simulink model "model"  (R2014a)
(part 3 of 3)

  _CN_133263110_220000_CN_163640749_220000/LConn3 -- T_133263110_220000_Няндома/LConn3 -- _CN_133263110_220000_CN_96836497_220000/LConn3 -- _CN_133263110_220000_CN_147416198_220000/LConn3 -- bus111/LConn1
  _CN_133263110_220000_CN_163640749_220000/RConn1 -- T_163640749_220000_Плесецк/LConn1 -- Плесецк___Новая_2_цепь_CN_163640749_220000_CN_124601500_220000/LConn1
  _CN_133263110_220000_CN_163640749_220000/RConn2 -- T_163640749_220000_Плесецк/LConn2 -- Плесецк___Новая_2_цепь_CN_163640749_220000_CN_124601500_220000/LConn2
  _CN_133263110_220000_CN_163640749_220000/RConn3 -- T_163640749_220000_Плесецк/LConn3 -- Плесецк___Новая_2_цепь_CN_163640749_220000_CN_124601500_220000/LConn3 -- bus112/LConn1
  _CN_133263110_220000_CN_96836497_220000/RConn1 -- T_96836497_220000_Коноша/LConn1 -- _CN_52300555_220000_CN_96836497_220000/LConn1
  _CN_133263110_220000_CN_96836497_220000/RConn2 -- T_96836497_220000_Коноша/LConn2 -- _CN_52300555_220000_CN_96836497_220000/LConn2
  _CN_133263110_220000_CN_96836497_220000/RConn3 -- T_96836497_220000_Коноша/LConn3 -- _CN_52300555_220000_CN_96836497_220000/LConn3 -- bus113/LConn1
  _CN_133263110_220000_CN_147416198_220000/RConn1 -- T_147416198_220000_Подстанция_220_кВ_«Вельск»/LConn1 -- Вельск___Шангалы_CN_147416198_220000_CN_265498319_220000/LConn1
  _CN_133263110_220000_CN_147416198_220000/RConn2 -- T_147416198_220000_Подстанция_220_кВ_«Вельск»/LConn2 -- Вельск___Шангалы_CN_147416198_220000_CN_265498319_220000/LConn2
  _CN_133263110_220000_CN_147416198_220000/RConn3 -- T_147416198_220000_Подстанция_220_кВ_«Вельск»/LConn3 -- Вельск___Шангалы_CN_147416198_220000_CN_265498319_220000/LConn3 -- bus114/LConn1
  _CN_52300555_220000_CN_331268073_220000/LConn1 -- "T_52300555__ПС_500кВ_\"Вологодская\""/LConn1 -- _CN_52300555_220000_CN_331298845_220000/LConn1 -- _CN_52300555_220000_CN_96836497_220000/RConn1 -- _CN_52300555_220000_CN_197906665_220000/LConn1 -- _CN_52300555_220000_CN_315281956_220000/LConn1
  _CN_52300555_220000_CN_331268073_220000/LConn2 -- "T_52300555__ПС_500кВ_\"Вологодская\""/LConn2 -- _CN_52300555_220000_CN_331298845_220000/LConn2 -- _CN_52300555_220000_CN_96836497_220000/RConn2 -- _CN_52300555_220000_CN_197906665_220000/LConn2 -- _CN_52300555_220000_CN_315281956_220000/LConn2
  _CN_52300555_220000_CN_331268073_220000/LConn3 -- "T_52300555__ПС_500кВ_\"Вологодская\""/LConn3 -- _CN_52300555_220000_CN_331298845_220000/LConn3 -- _CN_52300555_220000_CN_96836497_220000/RConn3 -- _CN_52300555_220000_CN_197906665_220000/LConn3 -- _CN_52300555_220000_CN_315281956_220000/LConn3 -- bus115/LConn1
  T_331268073_220000_ГПП_2/LConn1 -- _CN_52300555_220000_CN_331268073_220000/RConn1
  T_331268073_220000_ГПП_2/LConn2 -- _CN_52300555_220000_CN_331268073_220000/RConn2
  _CN_52300555_220000_CN_331268073_220000/RConn3 -- T_331268073_220000_ГПП_2/LConn3 -- bus116/LConn1
  T_331298845_220000_Явенга_тяговая/LConn1 -- _CN_52300555_220000_CN_331298845_220000/RConn1
  T_331298845_220000_Явенга_тяговая/LConn2 -- _CN_52300555_220000_CN_331298845_220000/RConn2
  _CN_52300555_220000_CN_331298845_220000/RConn3 -- T_331298845_220000_Явенга_тяговая/LConn3 -- bus117/LConn1
  T_197906665_220000_Кадниковский_тяговая/LConn1 -- _CN_52300555_220000_CN_197906665_220000/RConn1
  T_197906665_220000_Кадниковский_тяговая/LConn2 -- _CN_52300555_220000_CN_197906665_220000/RConn2
  _CN_52300555_220000_CN_197906665_220000/RConn3 -- T_197906665_220000_Кадниковский_тяговая/LConn3 -- bus118/LConn1
  T_315281956_220000_Сокол/LConn1 -- _CN_52300555_220000_CN_315281956_220000/RConn1
  T_315281956_220000_Сокол/LConn2 -- _CN_52300555_220000_CN_315281956_220000/RConn2
  _CN_52300555_220000_CN_315281956_220000/RConn3 -- T_315281956_220000_Сокол/LConn3 -- bus119/LConn1
  T_124601500_220000_Новая/LConn1 -- Плесецк___Новая_2_цепь_CN_163640749_220000_CN_124601500_220000/RConn1
  T_124601500_220000_Новая/LConn2 -- Плесецк___Новая_2_цепь_CN_163640749_220000_CN_124601500_220000/RConn2
  Плесецк___Новая_2_цепь_CN_163640749_220000_CN_124601500_220000/RConn3 -- T_124601500_220000_Новая/LConn3 -- bus120/LConn1
  Синдор___Микунь_CN_212471066_220000_CN_211036038_220000/RConn1 -- T_211036038_220000_Микунь/LConn1 -- _CN_276250552_220000_CN_211036038_220000/LConn1 -- Микунь___Сыктывкар_CN_217498367_220000_CN_211036038_220000/LConn1
  Синдор___Микунь_CN_212471066_220000_CN_211036038_220000/RConn2 -- T_211036038_220000_Микунь/LConn2 -- _CN_276250552_220000_CN_211036038_220000/LConn2 -- Микунь___Сыктывкар_CN_217498367_220000_CN_211036038_220000/LConn2
  Синдор___Микунь_CN_212471066_220000_CN_211036038_220000/RConn3 -- T_211036038_220000_Микунь/LConn3 -- _CN_276250552_220000_CN_211036038_220000/LConn3 -- Микунь___Сыктывкар_CN_217498367_220000_CN_211036038_220000/LConn3 -- bus121/LConn1
  "T_116869794_220000_Подстанция_\"Парголово\""/LConn1 -- _CN_116869794_220000_CN_23549613_220000/LConn1
  "T_116869794_220000_Подстанция_\"Парголово\""/LConn2 -- _CN_116869794_220000_CN_23549613_220000/LConn2
  _CN_116869794_220000_CN_23549613_220000/LConn3 -- "T_116869794_220000_Подстанция_\"Парголово\""/LConn3 -- bus122/LConn1
  "T_23549613_220000_Подстанция_\"Приморская\""/LConn1 -- _CN_116869794_220000_CN_23549613_220000/RConn1
  "T_23549613_220000_Подстанция_\"Приморская\""/LConn2 -- _CN_116869794_220000_CN_23549613_220000/RConn2
  _CN_116869794_220000_CN_23549613_220000/RConn3 -- "T_23549613_220000_Подстанция_\"Приморская\""/LConn3 -- bus123/LConn1
  T_105535524_220000_Промысловая/LConn1 -- Усинская___Промысловая_CN_105535524_220000_CN_105528914_220000/RConn1
  T_105535524_220000_Промысловая/LConn2 -- Усинская___Промысловая_CN_105535524_220000_CN_105528914_220000/RConn2
  Усинская___Промысловая_CN_105535524_220000_CN_105528914_220000/RConn3 -- T_105535524_220000_Промысловая/LConn3 -- bus124/LConn1
  Вельск___Шангалы_CN_147416198_220000_CN_265498319_220000/RConn1 -- T_265498319_220000_Шангалы/LConn1 -- Кизема__Шангалы_CN_163253148_220000_CN_265498319_220000/LConn1
  Вельск___Шангалы_CN_147416198_220000_CN_265498319_220000/RConn2 -- T_265498319_220000_Шангалы/LConn2 -- Кизема__Шангалы_CN_163253148_220000_CN_265498319_220000/LConn2
  Вельск___Шангалы_CN_147416198_220000_CN_265498319_220000/RConn3 -- T_265498319_220000_Шангалы/LConn3 -- Кизема__Шангалы_CN_163253148_220000_CN_265498319_220000/LConn3 -- bus125/LConn1
  Заовражье___Кизема_CN_163253148_220000_CN_159848384_220000/LConn1 -- T_163253148_220000_Подстанция_220_кВ_«Кизема»/LConn1 -- Кизема__Шангалы_CN_163253148_220000_CN_265498319_220000/RConn1
  Заовражье___Кизема_CN_163253148_220000_CN_159848384_220000/LConn2 -- T_163253148_220000_Подстанция_220_кВ_«Кизема»/LConn2 -- Кизема__Шангалы_CN_163253148_220000_CN_265498319_220000/RConn2
  Заовражье___Кизема_CN_163253148_220000_CN_159848384_220000/LConn3 -- T_163253148_220000_Подстанция_220_кВ_«Кизема»/LConn3 -- Кизема__Шангалы_CN_163253148_220000_CN_265498319_220000/RConn3 -- bus126/LConn1
  Заовражье___Кизема_CN_163253148_220000_CN_159848384_220000/RConn1 -- T_159848384_220000_Заовражье_1/LConn1 -- _CN_276250552_220000_CN_159848384_220000/LConn1
  Заовражье___Кизема_CN_163253148_220000_CN_159848384_220000/RConn2 -- T_159848384_220000_Заовражье_1/LConn2 -- _CN_276250552_220000_CN_159848384_220000/LConn2
  Заовражье___Кизема_CN_163253148_220000_CN_159848384_220000/RConn3 -- T_159848384_220000_Заовражье_1/LConn3 -- _CN_276250552_220000_CN_159848384_220000/LConn3 -- bus127/LConn1
  T_177805996_220000;110000;35000_ПС_220_кВ_Воркута/LConn1 -- ВЛ_220_кВ_Инта___Воркута_CN_177805996_220000_CN_88433653_220000/RConn1
  T_177805996_220000;110000;35000_ПС_220_кВ_Воркута/LConn2 -- ВЛ_220_кВ_Инта___Воркута_CN_177805996_220000_CN_88433653_220000/RConn2
  ВЛ_220_кВ_Инта___Воркута_CN_177805996_220000_CN_88433653_220000/RConn3 -- T_177805996_220000;110000;35000_ПС_220_кВ_Воркута/LConn3 -- bus128/LConn1
  T_260127849_220000_Газлифт/LConn1 -- _CN_260127849_220000_CN_105528914_220000/RConn1
  T_260127849_220000_Газлифт/LConn2 -- _CN_260127849_220000_CN_105528914_220000/RConn2
  _CN_260127849_220000_CN_105528914_220000/RConn3 -- T_260127849_220000_Газлифт/LConn3 -- bus129/LConn1
  _CN_276250552_220000_CN_211036038_220000/RConn1 -- T_276250552_220000_Урдома/LConn1 -- _CN_276250552_220000_CN_159848384_220000/RConn1
  _CN_276250552_220000_CN_211036038_220000/RConn2 -- T_276250552_220000_Урдома/LConn2 -- _CN_276250552_220000_CN_159848384_220000/RConn2
  _CN_276250552_220000_CN_211036038_220000/RConn3 -- T_276250552_220000_Урдома/LConn3 -- _CN_276250552_220000_CN_159848384_220000/RConn3 -- bus130/LConn1
  T_217498367_220000_Сыктывкар/LConn1 -- Микунь___Сыктывкар_CN_217498367_220000_CN_211036038_220000/RConn1
  T_217498367_220000_Сыктывкар/LConn2 -- Микунь___Сыктывкар_CN_217498367_220000_CN_211036038_220000/RConn2
  Микунь___Сыктывкар_CN_217498367_220000_CN_211036038_220000/RConn3 -- T_217498367_220000_Сыктывкар/LConn3 -- bus131/LConn1
  T_260124523_220000_Возейская/LConn1 -- Усинская___Возейская_CN_105528914_220000_CN_260124523_220000/RConn1
  T_260124523_220000_Возейская/LConn2 -- Усинская___Возейская_CN_105528914_220000_CN_260124523_220000/RConn2
  Усинская___Возейская_CN_105528914_220000_CN_260124523_220000/RConn3 -- T_260124523_220000_Возейская/LConn3 -- bus132/LConn1
  T_331932782_220000_КС_УГПЗ/LConn1 -- Усинская___КС_УГПЗ_CN_105528914_220000_CN_331932782_220000/RConn1
  T_331932782_220000_КС_УГПЗ/LConn2 -- Усинская___КС_УГПЗ_CN_105528914_220000_CN_331932782_220000/RConn2
  Усинская___КС_УГПЗ_CN_105528914_220000_CN_331932782_220000/RConn3 -- T_331932782_220000_КС_УГПЗ/LConn3 -- bus133/LConn1
  "T_202821548_330000;110000;10000_ПС_102_\"Великорецкая\"_330_110_10_кВ"/LConn1 -- _CN_202821548_330000_CN_201631421_330000/LConn1
  "T_202821548_330000;110000;10000_ПС_102_\"Великорецкая\"_330_110_10_кВ"/LConn2 -- _CN_202821548_330000_CN_201631421_330000/LConn2
  _CN_202821548_330000_CN_201631421_330000/LConn3 -- "T_202821548_330000;110000;10000_ПС_102_\"Великорецкая\"_330_110_10_кВ"/LConn3 -- bus134/LConn1
  _CN_202821548_330000_CN_201631421_330000/RConn1 -- T_201631421_330000;110000_ОРУ_330кВ/LConn1 -- _CN_34685101_330000_CN_201631421_330000/LConn1
  _CN_202821548_330000_CN_201631421_330000/RConn2 -- T_201631421_330000;110000_ОРУ_330кВ/LConn2 -- _CN_34685101_330000_CN_201631421_330000/LConn2
  _CN_202821548_330000_CN_201631421_330000/RConn3 -- T_201631421_330000;110000_ОРУ_330кВ/LConn3 -- _CN_34685101_330000_CN_201631421_330000/LConn3 -- bus135/LConn1
  _CN_357523602_330000_CN_89072244_330000/LConn1 -- T_357523602__/LConn1 -- _CN_357523602_330000_CN_47350956_330000/LConn1 -- _CN_357523602_330000_CN_302056096_330000/LConn1 -- _CN_357523602_330000_CN_125823925_330000/LConn1 -- _CN_357523602_330000_CN_100413661_330000/LConn1 -- _CN_357523602_330000_CN_87761736_330000/LConn1
  _CN_357523602_330000_CN_89072244_330000/LConn2 -- T_357523602__/LConn2 -- _CN_357523602_330000_CN_47350956_330000/LConn2 -- _CN_357523602_330000_CN_302056096_330000/LConn2 -- _CN_357523602_330000_CN_125823925_330000/LConn2 -- _CN_357523602_330000_CN_100413661_330000/LConn2 -- _CN_357523602_330000_CN_87761736_330000/LConn2
  _CN_357523602_330000_CN_89072244_330000/LConn3 -- T_357523602__/LConn3 -- _CN_357523602_330000_CN_47350956_330000/LConn3 -- bus136/LConn1 -- _CN_357523602_330000_CN_302056096_330000/LConn3 -- _CN_357523602_330000_CN_125823925_330000/LConn3 -- _CN_357523602_330000_CN_100413661_330000/LConn3 -- _CN_357523602_330000_CN_87761736_330000/LConn3
  T_89072244__ПС_Новгородская/LConn1 -- _CN_357523602_330000_CN_89072244_330000/RConn1
  T_89072244__ПС_Новгородская/LConn2 -- _CN_357523602_330000_CN_89072244_330000/RConn2
  _CN_357523602_330000_CN_89072244_330000/RConn3 -- T_89072244__ПС_Новгородская/LConn3 -- bus137/LConn1
  T_302056096__/LConn1 -- _CN_357523602_330000_CN_302056096_330000/RConn1
  T_302056096__/LConn2 -- _CN_357523602_330000_CN_302056096_330000/RConn2
  _CN_357523602_330000_CN_302056096_330000/RConn3 -- T_302056096__/LConn3 -- bus138/LConn1
  "T_125823925_330000_Подстация_\"Западная\""/LConn1 -- _CN_357523602_330000_CN_125823925_330000/RConn1
  "T_125823925_330000_Подстация_\"Западная\""/LConn2 -- _CN_357523602_330000_CN_125823925_330000/RConn2
  _CN_357523602_330000_CN_125823925_330000/RConn3 -- "T_125823925_330000_Подстация_\"Западная\""/LConn3 -- bus139/LConn1
  _CN_357523602_330000_CN_100413661_330000/RConn1 -- T_100413661_330000;110000;35000;6000_Гатчинская/LConn1 -- _CN_100413661_330000_CN_124275836_330000/LConn1
  _CN_357523602_330000_CN_100413661_330000/RConn2 -- T_100413661_330000;110000;35000;6000_Гатчинская/LConn2 -- _CN_100413661_330000_CN_124275836_330000/LConn2
  _CN_357523602_330000_CN_100413661_330000/RConn3 -- T_100413661_330000;110000;35000;6000_Гатчинская/LConn3 -- _CN_100413661_330000_CN_124275836_330000/LConn3 -- bus140/LConn1
  _CN_357523602_330000_CN_87761736_330000/RConn1 -- T_87761736_750000;330000;110000;10000_Ленинградская/LConn1 -- _CN_87761736_330000_CN_34682059_330000/LConn1 -- _CN_87761736_330000_CN_161733477_330000/LConn1
  _CN_357523602_330000_CN_87761736_330000/RConn2 -- T_87761736_750000;330000;110000;10000_Ленинградская/LConn2 -- _CN_87761736_330000_CN_34682059_330000/LConn2 -- _CN_87761736_330000_CN_161733477_330000/LConn2
  _CN_357523602_330000_CN_87761736_330000/RConn3 -- T_87761736_750000;330000;110000;10000_Ленинградская/LConn3 -- _CN_87761736_330000_CN_34682059_330000/LConn3 -- _CN_87761736_330000_CN_161733477_330000/LConn3 -- bus141/LConn1
  T_47350956__/LConn1 -- _CN_357523602_330000_CN_47350956_330000/RConn1
  T_47350956__/LConn2 -- _CN_357523602_330000_CN_47350956_330000/RConn2
  _CN_357523602_330000_CN_47350956_330000/RConn3 -- T_47350956__/LConn3 -- bus142/LConn1
  Калининградская_ТЭЦ_2_–_ПС_О_1_«Центральная»_CN_296188566_330000_CN_302938336_330000/LConn1 -- T_296188566_330000_ОРУ_330_кВ/LConn1 -- Калининградская_ТЭЦ_2_—_ПC_«Северная_330»_CN_296188566_330000_CN_53126382_330000/LConn1
  Калининградская_ТЭЦ_2_–_ПС_О_1_«Центральная»_CN_296188566_330000_CN_302938336_330000/LConn2 -- T_296188566_330000_ОРУ_330_кВ/LConn2 -- Калининградская_ТЭЦ_2_—_ПC_«Северная_330»_CN_296188566_330000_CN_53126382_330000/LConn2
  Калининградская_ТЭЦ_2_–_ПС_О_1_«Центральная»_CN_296188566_330000_CN_302938336_330000/LConn3 -- T_296188566_330000_ОРУ_330_кВ/LConn3 -- Калининградская_ТЭЦ_2_—_ПC_«Северная_330»_CN_296188566_330000_CN_53126382_330000/LConn3 -- bus143/LConn1
  Калининградская_ТЭЦ_2_–_ПС_О_1_«Центральная»_CN_296188566_330000_CN_302938336_330000/RConn1 -- T_302938336_330000;110000;15000_ПС_О_1_«Центральная»/LConn1 -- _CN_197911127_330000_CN_302938336_330000/LConn1
  Калининградская_ТЭЦ_2_–_ПС_О_1_«Центральная»_CN_296188566_330000_CN_302938336_330000/RConn2 -- T_302938336_330000;110000;15000_ПС_О_1_«Центральная»/LConn2 -- _CN_197911127_330000_CN_302938336_330000/LConn2
  Калининградская_ТЭЦ_2_–_ПС_О_1_«Центральная»_CN_296188566_330000_CN_302938336_330000/RConn3 -- T_302938336_330000;110000;15000_ПС_О_1_«Центральная»/LConn3 -- _CN_197911127_330000_CN_302938336_330000/LConn3 -- bus144/LConn1
  Калининградская_ТЭЦ_2_—_ПC_«Северная_330»_CN_296188566_330000_CN_53126382_330000/RConn1 -- T_53126382_330000;110000;15000_ПС_«Северная_330»/LConn1 -- _CN_197911127_330000_CN_53126382_330000/LConn1
  Калининградская_ТЭЦ_2_—_ПC_«Северная_330»_CN_296188566_330000_CN_53126382_330000/RConn2 -- T_53126382_330000;110000;15000_ПС_«Северная_330»/LConn2 -- _CN_197911127_330000_CN_53126382_330000/LConn2
  Калининградская_ТЭЦ_2_—_ПC_«Северная_330»_CN_296188566_330000_CN_53126382_330000/RConn3 -- T_53126382_330000;110000;15000_ПС_«Северная_330»/LConn3 -- _CN_197911127_330000_CN_53126382_330000/LConn3 -- bus145/LConn1
  _CN_285600732_330000_CN_25913909_330000/LConn1 -- T_285600732__/LConn1 -- _CN_285600732_330000_CN_24004349_330000/LConn1
  _CN_285600732_330000_CN_25913909_330000/LConn2 -- T_285600732__/LConn2 -- _CN_285600732_330000_CN_24004349_330000/LConn2
  _CN_285600732_330000_CN_25913909_330000/LConn3 -- T_285600732__/LConn3 -- _CN_285600732_330000_CN_24004349_330000/LConn3 -- bus146/LConn1
  _CN_285600732_330000_CN_25913909_330000/RConn1 -- "T_25913909_330000_Подстанция_\"Восточная\""/LConn1 -- _CN_25913909_330000_CN_197754700_330000/LConn1 -- _CN_25913909_330000_CN_55212134_330000/LConn1 -- _CN_25913909_330000_CN_161733477_330000/LConn1
  _CN_285600732_330000_CN_25913909_330000/RConn2 -- "T_25913909_330000_Подстанция_\"Восточная\""/LConn2 -- _CN_25913909_330000_CN_197754700_330000/LConn2 -- _CN_25913909_330000_CN_55212134_330000/LConn2 -- _CN_25913909_330000_CN_161733477_330000/LConn2
  _CN_285600732_330000_CN_25913909_330000/RConn3 -- "T_25913909_330000_Подстанция_\"Восточная\""/LConn3 -- _CN_25913909_330000_CN_197754700_330000/LConn3 -- _CN_25913909_330000_CN_55212134_330000/LConn3 -- _CN_25913909_330000_CN_161733477_330000/LConn3 -- bus147/LConn1
  "T_24004349_330000;110000;fixme_Подстанция_\"Северная\""/LConn1 -- _CN_285600732_330000_CN_24004349_330000/RConn1
  "T_24004349_330000;110000;fixme_Подстанция_\"Северная\""/LConn2 -- _CN_285600732_330000_CN_24004349_330000/RConn2
  _CN_285600732_330000_CN_24004349_330000/RConn3 -- "T_24004349_330000;110000;fixme_Подстанция_\"Северная\""/LConn3 -- bus148/LConn1
  _CN_34685101_330000_CN_124275836_330000/LConn1 -- T_34685101_330000_Eesti_EJ_alajaam/LConn1 -- _CN_34685101_330000_CN_201631421_330000/RConn1 -- _CN_34685101_330000_CN_34682059_330000/LConn1
  _CN_34685101_330000_CN_124275836_330000/LConn2 -- T_34685101_330000_Eesti_EJ_alajaam/LConn2 -- _CN_34685101_330000_CN_201631421_330000/RConn2 -- _CN_34685101_330000_CN_34682059_330000/LConn2
  _CN_34685101_330000_CN_124275836_330000/LConn3 -- T_34685101_330000_Eesti_EJ_alajaam/LConn3 -- _CN_34685101_330000_CN_201631421_330000/RConn3 -- _CN_34685101_330000_CN_34682059_330000/LConn3 -- bus149/LConn1
  _CN_34685101_330000_CN_124275836_330000/RConn1 -- T_124275836_330000;110000;fixme_ПС_Кингисеппская/LConn1 -- _CN_100413661_330000_CN_124275836_330000/RConn1
  _CN_34685101_330000_CN_124275836_330000/RConn2 -- T_124275836_330000;110000;fixme_ПС_Кингисеппская/LConn2 -- _CN_100413661_330000_CN_124275836_330000/RConn2
  _CN_34685101_330000_CN_124275836_330000/RConn3 -- T_124275836_330000;110000;fixme_ПС_Кингисеппская/LConn3 -- _CN_100413661_330000_CN_124275836_330000/RConn3 -- bus150/LConn1
  _CN_34685101_330000_CN_34682059_330000/RConn1 -- T_34682059_330000;110000_Balti_EJ_alajaam/LConn1 -- _CN_87761736_330000_CN_34682059_330000/RConn1 -- _CN_34682059_330000_CN_34682060_110000/RConn1
  _CN_34685101_330000_CN_34682059_330000/RConn2 -- T_34682059_330000;110000_Balti_EJ_alajaam/LConn2 -- _CN_87761736_330000_CN_34682059_330000/RConn2 -- _CN_34682059_330000_CN_34682060_110000/RConn2
  _CN_34685101_330000_CN_34682059_330000/RConn3 -- T_34682059_330000;110000_Balti_EJ_alajaam/LConn3 -- _CN_87761736_330000_CN_34682059_330000/RConn3 -- _CN_34682059_330000_CN_34682060_110000/RConn3 -- bus151/LConn1
  T_197754717__/LConn1 -- _CN_197754717_330000_CN_197754700_330000/LConn1
  T_197754717__/LConn2 -- _CN_197754717_330000_CN_197754700_330000/LConn2
  _CN_197754717_330000_CN_197754700_330000/LConn3 -- T_197754717__/LConn3 -- bus152/LConn1
  _CN_197754717_330000_CN_197754700_330000/RConn1 -- T_197754700__/LConn1 -- _CN_25913909_330000_CN_197754700_330000/RConn1 -- _CN_197754700_330000_CN_55212134_330000/LConn1
  _CN_197754717_330000_CN_197754700_330000/RConn2 -- T_197754700__/LConn2 -- _CN_25913909_330000_CN_197754700_330000/RConn2 -- _CN_197754700_330000_CN_55212134_330000/LConn2
  _CN_197754717_330000_CN_197754700_330000/RConn3 -- T_197754700__/LConn3 -- _CN_25913909_330000_CN_197754700_330000/RConn3 -- _CN_197754700_330000_CN_55212134_330000/LConn3 -- bus153/LConn1
  _CN_25913909_330000_CN_55212134_330000/RConn1 -- G_55212134_Киришская_ГРЭС/RConn1 -- _CN_197754700_330000_CN_55212134_330000/RConn1 -- _CN_169809022_330000_CN_55212134_330000/LConn1
  _CN_25913909_330000_CN_55212134_330000/RConn2 -- G_55212134_Киришская_ГРЭС/RConn2 -- _CN_197754700_330000_CN_55212134_330000/RConn2 -- _CN_169809022_330000_CN_55212134_330000/LConn2
  _CN_25913909_330000_CN_55212134_330000/RConn3 -- G_55212134_Киришская_ГРЭС/RConn3 -- _CN_197754700_330000_CN_55212134_330000/RConn3 -- _CN_169809022_330000_CN_55212134_330000/LConn3 -- bus154/LConn1
  _CN_25913909_330000_CN_161733477_330000/RConn1 -- "T_161733477_330000_Подстанция_\"Колпино\""/LConn1 -- _CN_87761736_330000_CN_161733477_330000/RConn1
  _CN_25913909_330000_CN_161733477_330000/RConn2 -- "T_161733477_330000_Подстанция_\"Колпино\""/LConn2 -- _CN_87761736_330000_CN_161733477_330000/RConn2
  _CN_25913909_330000_CN_161733477_330000/RConn3 -- "T_161733477_330000_Подстанция_\"Колпино\""/LConn3 -- _CN_87761736_330000_CN_161733477_330000/RConn3 -- bus155/LConn1
  _CN_197911127_330000_CN_53126382_330000/RConn1 -- T_197911127_330000;110000;15000;6000_ПС_330_кВ_«Советск»/LConn1 -- _CN_197911127_330000_CN_302938336_330000/RConn1
  _CN_197911127_330000_CN_53126382_330000/RConn2 -- T_197911127_330000;110000;15000;6000_ПС_330_кВ_«Советск»/LConn2 -- _CN_197911127_330000_CN_302938336_330000/RConn2
  _CN_197911127_330000_CN_53126382_330000/RConn3 -- T_197911127_330000;110000;15000;6000_ПС_330_кВ_«Советск»/LConn3 -- _CN_197911127_330000_CN_302938336_330000/RConn3 -- bus156/LConn1
  T_169809022__/LConn1 -- _CN_169809022_330000_CN_55212134_330000/RConn1
  T_169809022__/LConn2 -- _CN_169809022_330000_CN_55212134_330000/RConn2
  _CN_169809022_330000_CN_55212134_330000/RConn3 -- T_169809022__/LConn3 -- bus157/LConn1
  T_191502719__/LConn1 -- _CN_191502719_330000_CN_190866905_110000/RConn1
  T_191502719__/LConn2 -- _CN_191502719_330000_CN_190866905_110000/RConn2
  _CN_191502719_330000_CN_190866905_110000/RConn3 -- T_191502719__/LConn3 -- bus158/LConn1
  T_176029697__/RConn1 -- L_176029697/LConn1
  T_176029697__/RConn2 -- L_176029697/LConn2
  L_176029697/LConn3 -- T_176029697__/RConn3 -- bus159/LConn1
  T_279726507__ЭЧП_3/RConn1 -- L_279726507/LConn1
  T_279726507__ЭЧП_3/RConn2 -- L_279726507/LConn2
  L_279726507/LConn3 -- T_279726507__ЭЧП_3/RConn3 -- bus160/LConn1
  T_144555400__ЭЧП_5/RConn1 -- L_144555400/LConn1
  T_144555400__ЭЧП_5/RConn2 -- L_144555400/LConn2
  L_144555400/LConn3 -- T_144555400__ЭЧП_5/RConn3 -- bus161/LConn1
  T_184388878__Электростанция/RConn1 -- L_184388878/LConn1
  T_184388878__Электростанция/RConn2 -- L_184388878/LConn2
  L_184388878/LConn3 -- T_184388878__Электростанция/RConn3 -- bus162/LConn1
  T_200446426__/RConn1 -- L_200446426/LConn1
  T_200446426__/RConn2 -- L_200446426/LConn2
  L_200446426/LConn3 -- T_200446426__/RConn3 -- bus163/LConn1
  T_128423956__ЭПС_Мостищи_110_10_кВ/RConn1 -- L_128423956/LConn1
  T_128423956__ЭПС_Мостищи_110_10_кВ/RConn2 -- L_128423956/LConn2
  L_128423956/LConn3 -- T_128423956__ЭПС_Мостищи_110_10_кВ/RConn3 -- bus164/LConn1
  T_184189206__ЭПС_Базовая:_110_10_6_кВ/RConn1 -- L_184189206/LConn1
  T_184189206__ЭПС_Базовая:_110_10_6_кВ/RConn2 -- L_184189206/LConn2
  L_184189206/LConn3 -- T_184189206__ЭПС_Базовая:_110_10_6_кВ/RConn3 -- bus165/LConn1
  T_162611222__/RConn1 -- L_162611222/LConn1
  T_162611222__/RConn2 -- L_162611222/LConn2
  L_162611222/LConn3 -- T_162611222__/RConn3 -- bus166/LConn1
  T_164224743__/RConn1 -- L_164224743/LConn1
  T_164224743__/RConn2 -- L_164224743/LConn2
  L_164224743/LConn3 -- T_164224743__/RConn3 -- bus167/LConn1
  "T_139107864__Подстанция_\"Кораблестроительный_институт\""/RConn1 -- L_139107864/LConn1
  "T_139107864__Подстанция_\"Кораблестроительный_институт\""/RConn2 -- L_139107864/LConn2
  L_139107864/LConn3 -- "T_139107864__Подстанция_\"Кораблестроительный_институт\""/RConn3 -- bus168/LConn1
  T_87108350__/RConn1 -- L_87108350/LConn1
  T_87108350__/RConn2 -- L_87108350/LConn2
  L_87108350/LConn3 -- T_87108350__/RConn3 -- bus169/LConn1
  "T_160499737_110000;10000_ПС_399_\"ЭТЗ_Псков\"_110_10_кВ"/RConn1 -- L_160499737/LConn1
  "T_160499737_110000;10000_ПС_399_\"ЭТЗ_Псков\"_110_10_кВ"/RConn2 -- L_160499737/LConn2
  L_160499737/LConn3 -- "T_160499737_110000;10000_ПС_399_\"ЭТЗ_Псков\"_110_10_кВ"/RConn3 -- bus170/LConn1
  "T_114315616_110000;10000;6000_ПС_328_\"Заводская\"_110_10_6_кВ"/RConn1 -- L_114315616/LConn1
  "T_114315616_110000;10000;6000_ПС_328_\"Заводская\"_110_10_6_кВ"/RConn2 -- L_114315616/LConn2
  L_114315616/LConn3 -- "T_114315616_110000;10000;6000_ПС_328_\"Заводская\"_110_10_6_кВ"/RConn3 -- bus171/LConn1
  "T_135051666_110000;10000;6000_ПС_53_\"Псков\"_330_110_10_6_кВ"/RConn1 -- L_135051666/LConn1
  "T_135051666_110000;10000;6000_ПС_53_\"Псков\"_330_110_10_6_кВ"/RConn2 -- L_135051666/LConn2
  L_135051666/LConn3 -- "T_135051666_110000;10000;6000_ПС_53_\"Псков\"_330_110_10_6_кВ"/RConn3 -- bus172/LConn1
  "T_201631424_110000_ПС_126_\"Речная\"_110_6_кВ"/RConn1 -- L_201631424/LConn1
  "T_201631424_110000_ПС_126_\"Речная\"_110_6_кВ"/RConn2 -- L_201631424/LConn2
  L_201631424/LConn3 -- "T_201631424_110000_ПС_126_\"Речная\"_110_6_кВ"/RConn3 -- bus173/LConn1
  "T_126871068_110000;6000_ПС_73_\"Льнокомбинат\"_110_6_кВ"/RConn1 -- L_126871068/LConn1
  "T_126871068_110000;6000_ПС_73_\"Льнокомбинат\"_110_6_кВ"/RConn2 -- L_126871068/LConn2
  L_126871068/LConn3 -- "T_126871068_110000;6000_ПС_73_\"Льнокомбинат\"_110_6_кВ"/RConn3 -- bus174/LConn1
  "T_116910409_110000;10000_ПС_283_\"Завеличье\"_110_10_кВ"/RConn1 -- L_116910409/LConn1
  "T_116910409_110000;10000_ПС_283_\"Завеличье\"_110_10_кВ"/RConn2 -- L_116910409/LConn2
  L_116910409/LConn3 -- "T_116910409_110000;10000_ПС_283_\"Завеличье\"_110_10_кВ"/RConn3 -- bus175/LConn1
  T_202300588_110000_/RConn1 -- L_202300588/LConn1
  T_202300588_110000_/RConn2 -- L_202300588/LConn2
  L_202300588/LConn3 -- T_202300588_110000_/RConn3 -- bus176/LConn1
  "T_175342119__Подстанция_\"Невская_Дубровка\""/RConn1 -- L_175342119/LConn1
  "T_175342119__Подстанция_\"Невская_Дубровка\""/RConn2 -- L_175342119/LConn2
  L_175342119/LConn3 -- "T_175342119__Подстанция_\"Невская_Дубровка\""/RConn3 -- bus177/LConn1
  T_125089960__ПС_382_«Кировский_ЖБИ»/RConn1 -- L_125089960/LConn1
  T_125089960__ПС_382_«Кировский_ЖБИ»/RConn2 -- L_125089960/LConn2
  L_125089960/LConn3 -- T_125089960__ПС_382_«Кировский_ЖБИ»/RConn3 -- bus178/LConn1
  T_175342124__ПС_543_«Насосная»/RConn1 -- L_175342124/LConn1
  T_175342124__ПС_543_«Насосная»/RConn2 -- L_175342124/LConn2
  L_175342124/LConn3 -- T_175342124__ПС_543_«Насосная»/RConn3 -- bus179/LConn1
  T_160143087__ПС_555_«Невская»/RConn1 -- L_160143087/LConn1
  T_160143087__ПС_555_«Невская»/RConn2 -- L_160143087/LConn2
  L_160143087/LConn3 -- T_160143087__ПС_555_«Невская»/RConn3 -- bus180/LConn1
  "T_137274923__Подстанция_\"Парголово_Парнас\""/RConn1 -- L_137274923/LConn1
  "T_137274923__Подстанция_\"Парголово_Парнас\""/RConn2 -- L_137274923/LConn2
  L_137274923/LConn3 -- "T_137274923__Подстанция_\"Парголово_Парнас\""/RConn3 -- bus181/LConn1
  "T_79549681__Подстанция_\"Прядильно_ткацкая_фабрика\""/RConn1 -- L_79549681/LConn1
  "T_79549681__Подстанция_\"Прядильно_ткацкая_фабрика\""/RConn2 -- L_79549681/LConn2
  L_79549681/LConn3 -- "T_79549681__Подстанция_\"Прядильно_ткацкая_фабрика\""/RConn3 -- bus182/LConn1
  "T_108793849__Подстанция_\"Адамант\""/RConn1 -- L_108793849/LConn1
  "T_108793849__Подстанция_\"Адамант\""/RConn2 -- L_108793849/LConn2
  L_108793849/LConn3 -- "T_108793849__Подстанция_\"Адамант\""/RConn3 -- bus183/LConn1
  "T_74142253__Подстанция_\"Сосновская\""/RConn1 -- L_74142253/LConn1
  "T_74142253__Подстанция_\"Сосновская\""/RConn2 -- L_74142253/LConn2
  L_74142253/LConn3 -- "T_74142253__Подстанция_\"Сосновская\""/RConn3 -- bus184/LConn1
  "T_104487370__Подстация_\"Гражданская\""/RConn1 -- L_104487370/LConn1
  "T_104487370__Подстация_\"Гражданская\""/RConn2 -- L_104487370/LConn2
  L_104487370/LConn3 -- "T_104487370__Подстация_\"Гражданская\""/RConn3 -- bus185/LConn1
  T_142029975__ПС_№294_«Колтуши»/RConn1 -- L_142029975/LConn1
  T_142029975__ПС_№294_«Колтуши»/RConn2 -- L_142029975/LConn2
  L_142029975/LConn3 -- T_142029975__ПС_№294_«Колтуши»/RConn3 -- bus186/LConn1
  T_25452223__ПС_525_«Ильинка»/RConn1 -- L_25452223/LConn1
  T_25452223__ПС_525_«Ильинка»/RConn2 -- L_25452223/LConn2
  L_25452223/LConn3 -- T_25452223__ПС_525_«Ильинка»/RConn3 -- bus187/LConn1
  "T_142008798_110000_Трансформаторная_подстанция_\"Манушкино\""/RConn1 -- L_142008798/LConn1
  "T_142008798_110000_Трансформаторная_подстанция_\"Манушкино\""/RConn2 -- L_142008798/LConn2
  L_142008798/LConn3 -- "T_142008798_110000_Трансформаторная_подстанция_\"Манушкино\""/RConn3 -- bus188/LConn1
  "T_157742506__Подстанция_\"Янино\""/RConn1 -- L_157742506/LConn1
  "T_157742506__Подстанция_\"Янино\""/RConn2 -- L_157742506/LConn2
  L_157742506/LConn3 -- "T_157742506__Подстанция_\"Янино\""/RConn3 -- bus189/LConn1
  T_191152697__/RConn1 -- L_191152697/LConn1
  T_191152697__/RConn2 -- L_191152697/LConn2
  L_191152697/LConn3 -- T_191152697__/RConn3 -- bus190/LConn1
  T_191545113__/RConn1 -- L_191545113/LConn1
  T_191545113__/RConn2 -- L_191545113/LConn2
  L_191545113/LConn3 -- T_191545113__/RConn3 -- bus191/LConn1
  T_191152700__/RConn1 -- L_191152700/LConn1
  T_191152700__/RConn2 -- L_191152700/LConn2
  L_191152700/LConn3 -- T_191152700__/RConn3 -- bus192/LConn1
  T_191054670__/RConn1 -- L_191054670/LConn1
  T_191054670__/RConn2 -- L_191054670/LConn2
  L_191054670/LConn3 -- T_191054670__/RConn3 -- bus193/LConn1
  T_190857322__/RConn1 -- L_190857322/LConn1
  T_190857322__/RConn2 -- L_190857322/LConn2
  L_190857322/LConn3 -- T_190857322__/RConn3 -- bus194/LConn1
  T_188266306__/RConn1 -- L_188266306/LConn1
  T_188266306__/RConn2 -- L_188266306/LConn2
  L_188266306/LConn3 -- T_188266306__/RConn3 -- bus195/LConn1
  T_278548092__/RConn1 -- L_278548092/LConn1
  T_278548092__/RConn2 -- L_278548092/LConn2
  L_278548092/LConn3 -- T_278548092__/RConn3 -- bus196/LConn1
  T_278548104__/RConn1 -- L_278548104/LConn1
  T_278548104__/RConn2 -- L_278548104/LConn2
  L_278548104/LConn3 -- T_278548104__/RConn3 -- bus197/LConn1
  T_114922658_110000;35000;15000_/RConn1 -- L_114922658/LConn1
  T_114922658_110000;35000;15000_/RConn2 -- L_114922658/LConn2
  L_114922658/LConn3 -- T_114922658_110000;35000;15000_/RConn3 -- bus198/LConn1
  "T_162782315_110000;10000_ПС_110_10_№_66_\"Ломоносовская\""/RConn1 -- L_162782315/LConn1
  "T_162782315_110000;10000_ПС_110_10_№_66_\"Ломоносовская\""/RConn2 -- L_162782315/LConn2
  L_162782315/LConn3 -- "T_162782315_110000;10000_ПС_110_10_№_66_\"Ломоносовская\""/RConn3 -- bus199/LConn1
  T_165256814_110000;35000;10000_ПС_70_110_35_10_Жаровиха/RConn1 -- L_165256814/LConn1
  T_165256814_110000;35000;10000_ПС_70_110_35_10_Жаровиха/RConn2 -- L_165256814/LConn2
  L_165256814/LConn3 -- T_165256814_110000;35000;10000_ПС_70_110_35_10_Жаровиха/RConn3 -- bus200/LConn1
  T_345141892__/RConn1 -- L_345141892/LConn1
  T_345141892__/RConn2 -- L_345141892/LConn2
  L_345141892/LConn3 -- T_345141892__/RConn3 -- bus201/LConn1
  "T_46035010_220000_Подстанция_\"Колпинская\""/RConn1 -- L_46035010/LConn1
  "T_46035010_220000_Подстанция_\"Колпинская\""/RConn2 -- L_46035010/LConn2
  L_46035010/LConn3 -- "T_46035010_220000_Подстанция_\"Колпинская\""/RConn3 -- bus202/LConn1
  T_126367371__/RConn1 -- L_126367371/LConn1
  T_126367371__/RConn2 -- L_126367371/LConn2
  L_126367371/LConn3 -- T_126367371__/RConn3 -- bus203/LConn1
  T_230114987__ЭПС/RConn1 -- L_230114987/LConn1
  T_230114987__ЭПС/RConn2 -- L_230114987/LConn2
  L_230114987/LConn3 -- T_230114987__ЭПС/RConn3 -- bus204/LConn1
  T_206137484__ПС_43_«Гарболово»/RConn1 -- L_206137484/LConn1
  T_206137484__ПС_43_«Гарболово»/RConn2 -- L_206137484/LConn2
  L_206137484/LConn3 -- T_206137484__ПС_43_«Гарболово»/RConn3 -- bus205/LConn1
  T_205542778__ПС_47_«Лехтуси»/RConn1 -- L_205542778/LConn1
  T_205542778__ПС_47_«Лехтуси»/RConn2 -- L_205542778/LConn2
  L_205542778/LConn3 -- T_205542778__ПС_47_«Лехтуси»/RConn3 -- bus206/LConn1
  T_125115540_110000_/RConn1 -- L_125115540/LConn1
  T_125115540_110000_/RConn2 -- L_125115540/LConn2
  L_125115540/LConn3 -- T_125115540_110000_/RConn3 -- bus207/LConn1
  T_174003451__ПС_515_«ГПП_2»/RConn1 -- L_174003451/LConn1
  T_174003451__ПС_515_«ГПП_2»/RConn2 -- L_174003451/LConn2
  L_174003451/LConn3 -- T_174003451__ПС_515_«ГПП_2»/RConn3 -- bus208/LConn1
  T_153756310_110000;fixme_/RConn1 -- L_153756310/LConn1
  T_153756310_110000;fixme_/RConn2 -- L_153756310/LConn2
  L_153756310/LConn3 -- T_153756310_110000;fixme_/RConn3 -- bus209/LConn1
  T_179107625__/RConn1 -- L_179107625/LConn1
  T_179107625__/RConn2 -- L_179107625/LConn2
  L_179107625/LConn3 -- T_179107625__/RConn3 -- bus210/LConn1
  "T_27190951__ЭПС_\"Районная\""/RConn1 -- L_27190951/LConn1
  "T_27190951__ЭПС_\"Районная\""/RConn2 -- L_27190951/LConn2
  L_27190951/LConn3 -- "T_27190951__ЭПС_\"Районная\""/RConn3 -- bus211/LConn1
  T_356503018__/RConn1 -- L_356503018/LConn1
  T_356503018__/RConn2 -- L_356503018/LConn2
  L_356503018/LConn3 -- T_356503018__/RConn3 -- bus212/LConn1
  T_203028168_110000;fixme_/RConn1 -- L_203028168/LConn1
  T_203028168_110000;fixme_/RConn2 -- L_203028168/LConn2
  L_203028168/LConn3 -- T_203028168_110000;fixme_/RConn3 -- bus213/LConn1
  T_203028169_110000;fixme_/RConn1 -- L_203028169/LConn1
  T_203028169_110000;fixme_/RConn2 -- L_203028169/LConn2
  L_203028169/LConn3 -- T_203028169_110000;fixme_/RConn3 -- bus214/LConn1
  T_304918139_110000;35000;fixme_/RConn1 -- L_304918139/LConn1
  T_304918139_110000;35000;fixme_/RConn2 -- L_304918139/LConn2
  L_304918139/LConn3 -- T_304918139_110000;35000;fixme_/RConn3 -- bus215/LConn1
  T_152869732__Т_П_343_11/RConn1 -- L_152869732/LConn1
  T_152869732__Т_П_343_11/RConn2 -- L_152869732/LConn2
  L_152869732/LConn3 -- T_152869732__Т_П_343_11/RConn3 -- bus216/LConn1
  T_321829090_110000;10000_Joala_alajaam/RConn1 -- L_321829090/LConn1
  T_321829090_110000;10000_Joala_alajaam/RConn2 -- L_321829090/LConn2
  L_321829090/LConn3 -- T_321829090_110000;10000_Joala_alajaam/RConn3 -- bus217/LConn1
  T_35594708_110000;35000;6000_Narva_Peaalajaam/RConn1 -- L_35594708/LConn1
  T_35594708_110000;35000;6000_Narva_Peaalajaam/RConn2 -- L_35594708/LConn2
  L_35594708/LConn3 -- T_35594708_110000;35000;6000_Narva_Peaalajaam/RConn3 -- bus218/LConn1
  T_94121285_110000_Kreenholmi_alajaam/RConn1 -- L_94121285/LConn1
  T_94121285_110000_Kreenholmi_alajaam/RConn2 -- L_94121285/LConn2
  L_94121285/LConn3 -- T_94121285_110000_Kreenholmi_alajaam/RConn3 -- bus219/LConn1
  T_162207454__/RConn1 -- L_162207454/LConn1
  T_162207454__/RConn2 -- L_162207454/LConn2
  L_162207454/LConn3 -- T_162207454__/RConn3 -- bus220/LConn1
  T_125387022__/RConn1 -- L_125387022/LConn1
  T_125387022__/RConn2 -- L_125387022/LConn2
  L_125387022/LConn3 -- T_125387022__/RConn3 -- bus221/LConn1
  T_73882606__/RConn1 -- L_73882606/LConn1
  T_73882606__/RConn2 -- L_73882606/LConn2
  L_73882606/LConn3 -- T_73882606__/RConn3 -- bus222/LConn1
  T_55263465__Подстанция_№39/RConn1 -- L_55263465/LConn1
  T_55263465__Подстанция_№39/RConn2 -- L_55263465/LConn2
  L_55263465/LConn3 -- T_55263465__Подстанция_№39/RConn3 -- bus223/LConn1
  T_165278014__/RConn1 -- L_165278014/LConn1
  T_165278014__/RConn2 -- L_165278014/LConn2
  L_165278014/LConn3 -- T_165278014__/RConn3 -- bus224/LConn1
  T_95386425__ПС_№502_«Мартышкино»/RConn1 -- L_95386425/LConn1
  T_95386425__ПС_№502_«Мартышкино»/RConn2 -- L_95386425/LConn2
  L_95386425/LConn3 -- T_95386425__ПС_№502_«Мартышкино»/RConn3 -- bus225/LConn1
  T_95829467__Северная/RConn1 -- L_95829467/LConn1
  T_95829467__Северная/RConn2 -- L_95829467/LConn2
  L_95829467/LConn3 -- T_95829467__Северная/RConn3 -- bus226/LConn1
  T_152849205__ПС_403_«Мельничный_Ручей»/RConn1 -- L_152849205/LConn1
  T_152849205__ПС_403_«Мельничный_Ручей»/RConn2 -- L_152849205/LConn2
  L_152849205/LConn3 -- T_152849205__ПС_403_«Мельничный_Ручей»/RConn3 -- bus227/LConn1
  T_179043147__ПС_325_«Лепсари»/RConn1 -- L_179043147/LConn1
  T_179043147__ПС_325_«Лепсари»/RConn2 -- L_179043147/LConn2
  L_179043147/LConn3 -- T_179043147__ПС_325_«Лепсари»/RConn3 -- bus228/LConn1
  "T_205085439_110000;35000;10000_ПС_69_\"Изборск\"_110_35_10_кВ"/RConn1 -- L_205085439/LConn1
  "T_205085439_110000;35000;10000_ПС_69_\"Изборск\"_110_35_10_кВ"/RConn2 -- L_205085439/LConn2
  L_205085439/LConn3 -- "T_205085439_110000;35000;10000_ПС_69_\"Изборск\"_110_35_10_кВ"/RConn3 -- bus229/LConn1
  "T_205085437_110000_ПС_253_\"Тямша\"_110_10_кВ"/RConn1 -- L_205085437/LConn1
  "T_205085437_110000_ПС_253_\"Тямша\"_110_10_кВ"/RConn2 -- L_205085437/LConn2
  L_205085437/LConn3 -- "T_205085437_110000_ПС_253_\"Тямша\"_110_10_кВ"/RConn3 -- bus230/LConn1
  T_42675970_220000_Зашекснинская/RConn1 -- L_42675970/LConn1
  T_42675970_220000_Зашекснинская/RConn2 -- L_42675970/LConn2
  L_42675970/LConn3 -- T_42675970_220000_Зашекснинская/RConn3 -- bus231/LConn1
  T_328547675__/RConn1 -- L_328547675/LConn1
  T_328547675__/RConn2 -- L_328547675/LConn2
  L_328547675/LConn3 -- T_328547675__/RConn3 -- bus232/LConn1
  T_56029959__ПС_526_«Форд»/RConn1 -- L_56029959/LConn1
  T_56029959__ПС_526_«Форд»/RConn2 -- L_56029959/LConn2
  L_56029959/LConn3 -- T_56029959__ПС_526_«Форд»/RConn3 -- bus233/LConn1
  T_97385278__/RConn1 -- L_97385278/LConn1
  T_97385278__/RConn2 -- L_97385278/LConn2
  L_97385278/LConn3 -- T_97385278__/RConn3 -- bus234/LConn1
  T_302320627__/RConn1 -- L_302320627/LConn1
  T_302320627__/RConn2 -- L_302320627/LConn2
  L_302320627/LConn3 -- T_302320627__/RConn3 -- bus235/LConn1
  T_155145070__/RConn1 -- L_155145070/LConn1
  T_155145070__/RConn2 -- L_155145070/LConn2
  L_155145070/LConn3 -- T_155145070__/RConn3 -- bus236/LConn1
  T_289656575__/RConn1 -- L_289656575/LConn1
  T_289656575__/RConn2 -- L_289656575/LConn2
  L_289656575/LConn3 -- T_289656575__/RConn3 -- bus237/LConn1
  T_281578348__/RConn1 -- L_281578348/LConn1
  T_281578348__/RConn2 -- L_281578348/LConn2
  L_281578348/LConn3 -- T_281578348__/RConn3 -- bus238/LConn1
  T_321533904_110000;35000;fixme_/RConn1 -- L_321533904/LConn1
  T_321533904_110000;35000;fixme_/RConn2 -- L_321533904/LConn2
  L_321533904/LConn3 -- T_321533904_110000;35000;fixme_/RConn3 -- bus239/LConn1
  T_75305342__/RConn1 -- L_75305342/LConn1
  T_75305342__/RConn2 -- L_75305342/LConn2
  L_75305342/LConn3 -- T_75305342__/RConn3 -- bus240/LConn1
  "T_202389418_110000;10000_ПС_282_\"Овсище\"_110_10_кВ"/RConn1 -- L_202389418/LConn1
  "T_202389418_110000;10000_ПС_282_\"Овсище\"_110_10_кВ"/RConn2 -- L_202389418/LConn2
  L_202389418/LConn3 -- "T_202389418_110000;10000_ПС_282_\"Овсище\"_110_10_кВ"/RConn3 -- bus241/LConn1
  T_250170823_110000_/RConn1 -- L_250170823/LConn1
  T_250170823_110000_/RConn2 -- L_250170823/LConn2
  L_250170823/LConn3 -- T_250170823_110000_/RConn3 -- bus242/LConn1
  "T_175716081__ПС_100_\"Северная\"_110_10_кВ"/RConn1 -- L_175716081/LConn1
  "T_175716081__ПС_100_\"Северная\"_110_10_кВ"/RConn2 -- L_175716081/LConn2
  L_175716081/LConn3 -- "T_175716081__ПС_100_\"Северная\"_110_10_кВ"/RConn3 -- bus243/LConn1
  "T_252106171__ПС_110_кВ_\"Весьегонск\""/RConn1 -- L_252106171/LConn1
  "T_252106171__ПС_110_кВ_\"Весьегонск\""/RConn2 -- L_252106171/LConn2
  L_252106171/LConn3 -- "T_252106171__ПС_110_кВ_\"Весьегонск\""/RConn3 -- bus244/LConn1
  "T_252345291__ПС_110_кВ_\"Сандово\""/RConn1 -- L_252345291/LConn1
  "T_252345291__ПС_110_кВ_\"Сандово\""/RConn2 -- L_252345291/LConn2
  L_252345291/LConn3 -- "T_252345291__ПС_110_кВ_\"Сандово\""/RConn3 -- bus245/LConn1
  T_279665111_110000;15000_/RConn1 -- L_279665111/LConn1
  T_279665111_110000;15000_/RConn2 -- L_279665111/LConn2
  L_279665111/LConn3 -- T_279665111_110000;15000_/RConn3 -- bus246/LConn1
  "T_63107712_330000_Подстанция_\"Южная\""/RConn1 -- L_63107712/LConn1
  "T_63107712_330000_Подстанция_\"Южная\""/RConn2 -- L_63107712/LConn2
  L_63107712/LConn3 -- "T_63107712_330000_Подстанция_\"Южная\""/RConn3 -- bus247/LConn1
  T_87430145_220000_Печора/RConn1 -- L_87430145/LConn1
  T_87430145_220000_Печора/RConn2 -- L_87430145/LConn2
  L_87430145/LConn3 -- T_87430145_220000_Печора/RConn3 -- bus248/LConn1
  T_106941567_220000_Северная/RConn1 -- L_106941567/LConn1
  T_106941567_220000_Северная/RConn2 -- L_106941567/LConn2
  L_106941567/LConn3 -- T_106941567_220000_Северная/RConn3 -- bus249/LConn1
  T_88433653_220000;35000;10000_Инта_220/RConn1 -- L_88433653/LConn1
  T_88433653_220000;35000;10000_Инта_220/RConn2 -- L_88433653/LConn2
  L_88433653/LConn3 -- T_88433653_220000;35000;10000_Инта_220/RConn3 -- bus250/LConn1
  T_105528914_220000_Усинская/RConn1 -- L_105528914/LConn1
  T_105528914_220000_Усинская/RConn2 -- L_105528914/LConn2
  L_105528914/LConn3 -- T_105528914_220000_Усинская/RConn3 -- bus251/LConn1
  "T_152126979_220000_ПС_220_кВ_\"Ухта\""/RConn1 -- L_152126979/LConn1
  "T_152126979_220000_ПС_220_кВ_\"Ухта\""/RConn2 -- L_152126979/LConn2
  L_152126979/LConn3 -- "T_152126979_220000_ПС_220_кВ_\"Ухта\""/RConn3 -- bus252/LConn1
  T_212471066_220000_Синдор/RConn1 -- L_212471066/LConn1
  T_212471066_220000_Синдор/RConn2 -- L_212471066/LConn2
  L_212471066/LConn3 -- T_212471066_220000_Синдор/RConn3 -- bus253/LConn1
  T_133263110_220000_Няндома/RConn1 -- L_133263110/LConn1
  T_133263110_220000_Няндома/RConn2 -- L_133263110/LConn2
  L_133263110/LConn3 -- T_133263110_220000_Няндома/RConn3 -- bus254/LConn1
  T_163640749_220000_Плесецк/RConn1 -- L_163640749/LConn1
  T_163640749_220000_Плесецк/RConn2 -- L_163640749/LConn2
  L_163640749/LConn3 -- T_163640749_220000_Плесецк/RConn3 -- bus255/LConn1
  T_96836497_220000_Коноша/RConn1 -- L_96836497/LConn1
  T_96836497_220000_Коноша/RConn2 -- L_96836497/LConn2
  L_96836497/LConn3 -- T_96836497_220000_Коноша/RConn3 -- bus256/LConn1
  T_147416198_220000_Подстанция_220_кВ_«Вельск»/RConn1 -- L_147416198/LConn1
  T_147416198_220000_Подстанция_220_кВ_«Вельск»/RConn2 -- L_147416198/LConn2
  L_147416198/LConn3 -- T_147416198_220000_Подстанция_220_кВ_«Вельск»/RConn3 -- bus257/LConn1
  "T_52300555__ПС_500кВ_\"Вологодская\""/RConn1 -- L_52300555/LConn1
  "T_52300555__ПС_500кВ_\"Вологодская\""/RConn2 -- L_52300555/LConn2
  L_52300555/LConn3 -- "T_52300555__ПС_500кВ_\"Вологодская\""/RConn3 -- bus258/LConn1
  T_331268073_220000_ГПП_2/RConn1 -- L_331268073/LConn1
  T_331268073_220000_ГПП_2/RConn2 -- L_331268073/LConn2
  L_331268073/LConn3 -- T_331268073_220000_ГПП_2/RConn3 -- bus259/LConn1
  T_331298845_220000_Явенга_тяговая/RConn1 -- L_331298845/LConn1
  T_331298845_220000_Явенга_тяговая/RConn2 -- L_331298845/LConn2
  L_331298845/LConn3 -- T_331298845_220000_Явенга_тяговая/RConn3 -- bus260/LConn1
  T_197906665_220000_Кадниковский_тяговая/RConn1 -- L_197906665/LConn1
  T_197906665_220000_Кадниковский_тяговая/RConn2 -- L_197906665/LConn2
  L_197906665/LConn3 -- T_197906665_220000_Кадниковский_тяговая/RConn3 -- bus261/LConn1
  T_315281956_220000_Сокол/RConn1 -- L_315281956/LConn1
  T_315281956_220000_Сокол/RConn2 -- L_315281956/LConn2
  L_315281956/LConn3 -- T_315281956_220000_Сокол/RConn3 -- bus262/LConn1
  T_124601500_220000_Новая/RConn1 -- L_124601500/LConn1
  T_124601500_220000_Новая/RConn2 -- L_124601500/LConn2
  L_124601500/LConn3 -- T_124601500_220000_Новая/RConn3 -- bus263/LConn1
  T_211036038_220000_Микунь/RConn1 -- L_211036038/LConn1
  T_211036038_220000_Микунь/RConn2 -- L_211036038/LConn2
  L_211036038/LConn3 -- T_211036038_220000_Микунь/RConn3 -- bus264/LConn1
  "T_116869794_220000_Подстанция_\"Парголово\""/RConn1 -- L_116869794/LConn1
  "T_116869794_220000_Подстанция_\"Парголово\""/RConn2 -- L_116869794/LConn2
  L_116869794/LConn3 -- "T_116869794_220000_Подстанция_\"Парголово\""/RConn3 -- bus265/LConn1
  "T_23549613_220000_Подстанция_\"Приморская\""/RConn1 -- L_23549613/LConn1
  "T_23549613_220000_Подстанция_\"Приморская\""/RConn2 -- L_23549613/LConn2
  L_23549613/LConn3 -- "T_23549613_220000_Подстанция_\"Приморская\""/RConn3 -- bus266/LConn1
  T_105535524_220000_Промысловая/RConn1 -- L_105535524/LConn1
  T_105535524_220000_Промысловая/RConn2 -- L_105535524/LConn2
  L_105535524/LConn3 -- T_105535524_220000_Промысловая/RConn3 -- bus267/LConn1
  T_265498319_220000_Шангалы/RConn1 -- L_265498319/LConn1
  T_265498319_220000_Шангалы/RConn2 -- L_265498319/LConn2
  L_265498319/LConn3 -- T_265498319_220000_Шангалы/RConn3 -- bus268/LConn1
  T_163253148_220000_Подстанция_220_кВ_«Кизема»/RConn1 -- L_163253148/LConn1
  T_163253148_220000_Подстанция_220_кВ_«Кизема»/RConn2 -- L_163253148/LConn2
  L_163253148/LConn3 -- T_163253148_220000_Подстанция_220_кВ_«Кизема»/RConn3 -- bus269/LConn1
  T_159848384_220000_Заовражье_1/RConn1 -- L_159848384/LConn1
  T_159848384_220000_Заовражье_1/RConn2 -- L_159848384/LConn2
  L_159848384/LConn3 -- T_159848384_220000_Заовражье_1/RConn3 -- bus270/LConn1
  T_177805996_220000;110000;35000_ПС_220_кВ_Воркута/RConn1 -- L_177805996/LConn1
  T_177805996_220000;110000;35000_ПС_220_кВ_Воркута/RConn2 -- L_177805996/LConn2
  L_177805996/LConn3 -- T_177805996_220000;110000;35000_ПС_220_кВ_Воркута/RConn3 -- bus271/LConn1
  T_260127849_220000_Газлифт/RConn1 -- L_260127849/LConn1
  T_260127849_220000_Газлифт/RConn2 -- L_260127849/LConn2
  L_260127849/LConn3 -- T_260127849_220000_Газлифт/RConn3 -- bus272/LConn1
  T_276250552_220000_Урдома/RConn1 -- L_276250552/LConn1
  T_276250552_220000_Урдома/RConn2 -- L_276250552/LConn2
  L_276250552/LConn3 -- T_276250552_220000_Урдома/RConn3 -- bus273/LConn1
  T_217498367_220000_Сыктывкар/RConn1 -- L_217498367/LConn1
  T_217498367_220000_Сыктывкар/RConn2 -- L_217498367/LConn2
  L_217498367/LConn3 -- T_217498367_220000_Сыктывкар/RConn3 -- bus274/LConn1
  T_260124523_220000_Возейская/RConn1 -- L_260124523/LConn1
  T_260124523_220000_Возейская/RConn2 -- L_260124523/LConn2
  L_260124523/LConn3 -- T_260124523_220000_Возейская/RConn3 -- bus275/LConn1
  T_331932782_220000_КС_УГПЗ/RConn1 -- L_331932782/LConn1
  T_331932782_220000_КС_УГПЗ/RConn2 -- L_331932782/LConn2
  L_331932782/LConn3 -- T_331932782_220000_КС_УГПЗ/RConn3 -- bus276/LConn1
  "T_202821548_330000;110000;10000_ПС_102_\"Великорецкая\"_330_110_10_кВ"/RConn1 -- L_202821548/LConn1
  "T_202821548_330000;110000;10000_ПС_102_\"Великорецкая\"_330_110_10_кВ"/RConn2 -- L_202821548/LConn2
  L_202821548/LConn3 -- "T_202821548_330000;110000;10000_ПС_102_\"Великорецкая\"_330_110_10_кВ"/RConn3 -- bus277/LConn1
  T_201631421_330000;110000_ОРУ_330кВ/RConn1 -- L_201631421/LConn1
  T_201631421_330000;110000_ОРУ_330кВ/RConn2 -- L_201631421/LConn2
  L_201631421/LConn3 -- T_201631421_330000;110000_ОРУ_330кВ/RConn3 -- bus278/LConn1
  T_357523602__/RConn1 -- L_357523602/LConn1
  T_357523602__/RConn2 -- L_357523602/LConn2
  L_357523602/LConn3 -- T_357523602__/RConn3 -- bus279/LConn1
  T_89072244__ПС_Новгородская/RConn1 -- L_89072244/LConn1
  T_89072244__ПС_Новгородская/RConn2 -- L_89072244/LConn2
  L_89072244/LConn3 -- T_89072244__ПС_Новгородская/RConn3 -- bus280/LConn1
  T_302056096__/RConn1 -- L_302056096/LConn1
  T_302056096__/RConn2 -- L_302056096/LConn2
  L_302056096/LConn3 -- T_302056096__/RConn3 -- bus281/LConn1
  T_100413661_330000;110000;35000;6000_Гатчинская/RConn1 -- L_100413661/LConn1
  T_100413661_330000;110000;35000;6000_Гатчинская/RConn2 -- L_100413661/LConn2
  L_100413661/LConn3 -- T_100413661_330000;110000;35000;6000_Гатчинская/RConn3 -- bus282/LConn1
  T_87761736_750000;330000;110000;10000_Ленинградская/RConn1 -- L_87761736/LConn1
  T_87761736_750000;330000;110000;10000_Ленинградская/RConn2 -- L_87761736/LConn2
  L_87761736/LConn3 -- T_87761736_750000;330000;110000;10000_Ленинградская/RConn3 -- bus283/LConn1
  T_47350956__/RConn1 -- L_47350956/LConn1
  T_47350956__/RConn2 -- L_47350956/LConn2
  L_47350956/LConn3 -- T_47350956__/RConn3 -- bus284/LConn1
  T_296188566_330000_ОРУ_330_кВ/RConn1 -- L_296188566/LConn1
  T_296188566_330000_ОРУ_330_кВ/RConn2 -- L_296188566/LConn2
  L_296188566/LConn3 -- T_296188566_330000_ОРУ_330_кВ/RConn3 -- bus285/LConn1
  T_285600732__/RConn1 -- L_285600732/LConn1
  T_285600732__/RConn2 -- L_285600732/LConn2
  L_285600732/LConn3 -- T_285600732__/RConn3 -- bus286/LConn1
  T_34685101_330000_Eesti_EJ_alajaam/RConn1 -- L_34685101/LConn1
  T_34685101_330000_Eesti_EJ_alajaam/RConn2 -- L_34685101/LConn2
  L_34685101/LConn3 -- T_34685101_330000_Eesti_EJ_alajaam/RConn3 -- bus287/LConn1
  T_124275836_330000;110000;fixme_ПС_Кингисеппская/RConn1 -- L_124275836/LConn1
  T_124275836_330000;110000;fixme_ПС_Кингисеппская/RConn2 -- L_124275836/LConn2
  L_124275836/LConn3 -- T_124275836_330000;110000;fixme_ПС_Кингисеппская/RConn3 -- bus288/LConn1
  T_197754717__/RConn1 -- L_197754717/LConn1
  T_197754717__/RConn2 -- L_197754717/LConn2
  L_197754717/LConn3 -- T_197754717__/RConn3 -- bus289/LConn1
  T_197754700__/RConn1 -- L_197754700/LConn1
  T_197754700__/RConn2 -- L_197754700/LConn2
  L_197754700/LConn3 -- T_197754700__/RConn3 -- bus290/LConn1
  T_197911127_330000;110000;15000;6000_ПС_330_кВ_«Советск»/RConn1 -- L_197911127/LConn1
  T_197911127_330000;110000;15000;6000_ПС_330_кВ_«Советск»/RConn2 -- L_197911127/LConn2
  L_197911127/LConn3 -- T_197911127_330000;110000;15000;6000_ПС_330_кВ_«Советск»/RConn3 -- bus291/LConn1
